simulink model "batteryModel"  (R2022b)
settings: Solver=VariableStepAuto  StartTime=0.0  StopTime=80000  RelTol=1e-3
PreLoadFcn:
  | first_run_this_to_import_nedc_data
  | batteryModel_ini
InitFcn:
  | first_run_this_to_import_nedc_data
  | batteryModel_ini
values from neighbouring files (symbols this model uses):
  Battery =     [BatteryParameters.mat]
  I = [1.29210780767e-28 1.29210780767e-28 1.29210780767e-28 1.29210780767e-28 1.29210780767e-28 1.29210780767e-28 1.29210780767e-28 1.29210780767e-28 1.29210780767e-28 1.29210780767e-28 1.29210780767e-28 4.77614030937 ... (41369 elements, 41369x1)]    [BatteryParameters.mat]
  OCVSOC = [2 2 0.95 1.1 0.95 0.79 1.02 0.92 0.75 0.87]    [BatteryParameters.mat]    (also in OCVSOC.mat)
  Ts = 1    [BatteryParameters.mat]    (also in myFunction.m; test1.m)
undefined symbols (not defined in the file or in its folder): sigbuilder_block
libraries: neural x50, fl_lib x7, nesl_utility x6, dspstat3 x3, simulink x2, sharedTrackingLibrary x2, batteryecm_lib x1, ctrlSharedLib x1
(part 3 of 3)

== matlab function batteryModel/UKF/Simulink Function - State Transition Function/f(x,u) ==
  data: x input; R1 input; R2 input; R3 input; t1 input; t2 input; t3 input; Cq input; I input; xdot output
function xdot = fx(x,R1,R2,R3,t1,t2,t3,Cq,I)
xdot = zeros(size(x));
U1 = x(2);
U2 = x(3);
U3 = x(4);
xdot(1) = -I/(3600*Cq);
xdot(2) = -1/t1*U1 + I/(t1/R1);
xdot(3) = -1/t2*U2 + I/(t2/R2);
xdot(4) = -1/t3*U3 + I/(t3/R3);
xdot(5) = 0;

== matlab function batteryModel/EKF/Simulink Function - State Transition Function/f(x,u) ==
  data: x input; R1 input; R2 input; R3 input; t1 input; t2 input; t3 input; Cq input; I input; xdot output
function xdot = fx(x,R1,R2,R3,t1,t2,t3,Cq,I)
xdot = zeros(size(x));
U1 = x(2);
U2 = x(3);
U3 = x(4);
xdot(1) = -I/(3600*Cq);
xdot(2) = -1/t1*U1 + I/(t1/R1);
xdot(3) = -1/t2*U2 + I/(t2/R2);
xdot(4) = -1/t3*U3 + I/(t3/R3);
xdot(5) = 0;

== matlab function batteryModel/EKF/MATLAB Function ==
  data: V input; SOC_Estimated output; I input; T input; Vt_Estimated output; Vt_Error output; Xk input; Xk1 output; R0 input; R1 input; Tau1 input; OCV input; P_x input; P_x1 output; Q_x input; R_x input; Q_x1 output; R_x1 output; V1 output; KalmanGain_x output; Docv_soc input
function [SOC_Estimated, Vt_Estimated, Vt_Error, Xk1, P_x1, Q_x1,R_x1,V1,KalmanGain_x] = fcn(V, I, T, Xk, R0, R1,Tau1 ,OCV, P_x, Q_x, R_x, Docv_soc)

%comment for AEKF
 Q_x = [1.0e-10 0;0 1.0e-10];
 R_x   = 1;

n_x   = size(Xk,1);

DeltaT = 1;

Qn_rated    = 5 * 3600; % Ah to Amp-seconds

SOC = Xk(1);
V1 = Xk(2);

Tau_1 = Tau1;
    
a1 = exp(-DeltaT/Tau_1);
    
b1 = R1 * (1 - exp(-DeltaT/Tau_1));

    
TerminalVoltage = OCV - R0*I - V1;  

C_x    = [Docv_soc -1];

Error_x   = V - TerminalVoltage;
    
Vt_Estimated = TerminalVoltage;
SOC_Estimated = Xk(1);

Vt_Error = Error_x;

    
    A   = [1 0;
           0 a1];

    B   = [-(DeltaT/Qn_rated); b1];

    Xk   = (A * Xk) + (B * I);
    P_x = (A * P_x * A') + Q_x;
    
    KalmanGain_x = (P_x) * (C_x') * (inv((C_x * P_x * C_x') + (R_x)));
    Xk1 = Xk + (KalmanGain_x * Error_x);
    P_x1 = (eye(n_x,n_x) - (KalmanGain_x * C_x)) * P_x;
    
   
    %adaptive ekf (aekf)
    Q_x1 = KalmanGain_x * Error_x * KalmanGain_x';
    R_x1 = Error_x - C_x * P_x * C_x';



    %y = [SOC_Estimated, Vt_Estimated, Vt_Error, Xk1, P_x1];
